simulink library "TYPEBP_MASTER"  (Simulink 8.6)
settings: Solver=ode45  StartTime=0.0  StopTime=10.0  RelTol=1e-3
undefined symbols (not defined in the file): TYPEC, TYPEC_MASTER
libraries: cdsEpicsOut x38, cdsFilt x34, cdsFiltCtrl x24, STATE_BIO_MASTER x18, cdsTP x16, cdsEpicsBinIn x9, VIS_LIB x8, cdsEpicsIn x8, cdsMuxMatrix x5, SIXOSEM_F_STAGE_MASTER x4, cdsEpicsStringIn x3, cdsDacKill x3
(part 2 of 8)

== system TYPEBP_MASTER/TYPEBPMASTER/TEST ==
  In1 : Inport
  In4 : Inport  Port=2
  In7 : Inport  Port=3
  In10 : Inport  Port=4
  CH1 : cdsFiltCtrl/IIR FM with control  Tag=cdsFiltCtrl  Description=|
      | cdsFiltCntrl is the standard IIR filter module (exactly the same as cdsFilt) but with added control data output 'Ctrl'. Filter module digital signal output appears on the first output, which is called 'Val'. 'Ctrl' output has a bit pattern encoding the state of filter's on/off switches (FM1 through FM10). The bit values are:
      |                                                                                                                                                                                                                                                                                                                                       
      | module 	hex	dec                                                                                                                                                                                                                                                                                                                       
      | -----------------------                                                                                                                                                                                                                                                                                                               
      | FM1	0x20                    32                                                                                                                                                                                                                                                                                                        
      | FM2	0x80                     128                                                                                                                                                                                                                                                                                                      
      | FM3	0x200                   512                                                                                                                                                                                                                                                                                                       
      | FM4	0x800                   2048                                                                                                                                                                                                                                                                                                      
      | FM5	0x2000                 8192                                                                                                                                                                                                                                                                                                       
      | FM6	0x8000                 32768                                                                                                                                                                                                                                                                                                      
      | FM7	0x20000                131072                                                                                                                                                                                                                                                                                                     
      | FM8	0x80000                 524288                                                                                                                                                                                                                                                                                                    
      | FM9	0x200000               2097152                                                                                                                                                                                                                                                                                                    
      | FM10	0x800000               8388608                                                                                                                                                                                                                                                                                                   
      |                                                                                                                                                                                                                                                                                                                                       
      | This bit data can be used to drive some other switches or it can be output using a binary I/O module.
      settings: AttributesFormatString=%<Tag>
  CH2 : cdsFiltCtrl/IIR FM with control  Tag=cdsFiltCtrl  Description=|
      | cdsFiltCntrl is the standard IIR filter module (exactly the same as cdsFilt) but with added control data output 'Ctrl'. Filter module digital signal output appears on the first output, which is called 'Val'. 'Ctrl' output has a bit pattern encoding the state of filter's on/off switches (FM1 through FM10). The bit values are:
      |                                                                                                                                                                                                                                                                                                                                       
      | module 	hex	dec                                                                                                                                                                                                                                                                                                                       
      | -----------------------                                                                                                                                                                                                                                                                                                               
      | FM1	0x20                    32                                                                                                                                                                                                                                                                                                        
      | FM2	0x80                     128                                                                                                                                                                                                                                                                                                      
      | FM3	0x200                   512                                                                                                                                                                                                                                                                                                       
      | FM4	0x800                   2048                                                                                                                                                                                                                                                                                                      
      | FM5	0x2000                 8192                                                                                                                                                                                                                                                                                                       
      | FM6	0x8000                 32768                                                                                                                                                                                                                                                                                                      
      | FM7	0x20000                131072                                                                                                                                                                                                                                                                                                     
      | FM8	0x80000                 524288                                                                                                                                                                                                                                                                                                    
      | FM9	0x200000               2097152                                                                                                                                                                                                                                                                                                    
      | FM10	0x800000               8388608                                                                                                                                                                                                                                                                                                   
      |                                                                                                                                                                                                                                                                                                                                       
      | This bit data can be used to drive some other switches or it can be output using a binary I/O module.
      settings: AttributesFormatString=%<Tag>
  CH3 : cdsFiltCtrl/IIR FM with control  Tag=cdsFiltCtrl  Description=|
      | cdsFiltCntrl is the standard IIR filter module (exactly the same as cdsFilt) but with added control data output 'Ctrl'. Filter module digital signal output appears on the first output, which is called 'Val'. 'Ctrl' output has a bit pattern encoding the state of filter's on/off switches (FM1 through FM10). The bit values are:
      |                                                                                                                                                                                                                                                                                                                                       
      | module 	hex	dec                                                                                                                                                                                                                                                                                                                       
      | -----------------------                                                                                                                                                                                                                                                                                                               
      | FM1	0x20                    32                                                                                                                                                                                                                                                                                                        
      | FM2	0x80                     128                                                                                                                                                                                                                                                                                                      
      | FM3	0x200                   512                                                                                                                                                                                                                                                                                                       
      | FM4	0x800                   2048                                                                                                                                                                                                                                                                                                      
      | FM5	0x2000                 8192                                                                                                                                                                                                                                                                                                       
      | FM6	0x8000                 32768                                                                                                                                                                                                                                                                                                      
      | FM7	0x20000                131072                                                                                                                                                                                                                                                                                                     
      | FM8	0x80000                 524288                                                                                                                                                                                                                                                                                                    
      | FM9	0x200000               2097152                                                                                                                                                                                                                                                                                                    
      | FM10	0x800000               8388608                                                                                                                                                                                                                                                                                                   
      |                                                                                                                                                                                                                                                                                                                                       
      | This bit data can be used to drive some other switches or it can be output using a binary I/O module.
      settings: AttributesFormatString=%<Tag>
  CH4 : cdsFiltCtrl/IIR FM with control  Tag=cdsFiltCtrl  Description=|
      | cdsFiltCntrl is the standard IIR filter module (exactly the same as cdsFilt) but with added control data output 'Ctrl'. Filter module digital signal output appears on the first output, which is called 'Val'. 'Ctrl' output has a bit pattern encoding the state of filter's on/off switches (FM1 through FM10). The bit values are:
      |                                                                                                                                                                                                                                                                                                                                       
      | module 	hex	dec                                                                                                                                                                                                                                                                                                                       
      | -----------------------                                                                                                                                                                                                                                                                                                               
      | FM1	0x20                    32                                                                                                                                                                                                                                                                                                        
      | FM2	0x80                     128                                                                                                                                                                                                                                                                                                      
      | FM3	0x200                   512                                                                                                                                                                                                                                                                                                       
      | FM4	0x800                   2048                                                                                                                                                                                                                                                                                                      
      | FM5	0x2000                 8192                                                                                                                                                                                                                                                                                                       
      | FM6	0x8000                 32768                                                                                                                                                                                                                                                                                                      
      | FM7	0x20000                131072                                                                                                                                                                                                                                                                                                     
      | FM8	0x80000                 524288                                                                                                                                                                                                                                                                                                    
      | FM9	0x200000               2097152                                                                                                                                                                                                                                                                                                    
      | FM10	0x800000               8388608                                                                                                                                                                                                                                                                                                   
      |                                                                                                                                                                                                                                                                                                                                       
      | This bit data can be used to drive some other switches or it can be output using a binary I/O module.
      settings: AttributesFormatString=%<Tag>
  Ground{1..6,19,22} (8 alike) : Ground
  Terminator{1..5,16..18} (8 alike) : Terminator
  wires:
  CH1/1 -> Terminator5/1
  CH3/1 -> Terminator3/1
  CH4/1 -> Terminator2/1
  In4/1 -> CH2/1
  CH2/1 -> Terminator4/1
  In1/1 -> CH1/1
  In7/1 -> CH3/1
  In10/1 -> CH4/1
  Ground22/1 -> CH1/2
  Ground19/1 -> CH1/3
  CH1/2 -> Terminator16/1
  CH2/2 -> Terminator17/1
  CH3/2 -> Terminator18/1
  Ground2/1 -> CH2/2
  Ground1/1 -> CH2/3
  Ground4/1 -> CH3/2
  Ground3/1 -> CH3/3
  Ground6/1 -> CH4/2
  Ground5/1 -> CH4/3
  CH4/2 -> Terminator1/1

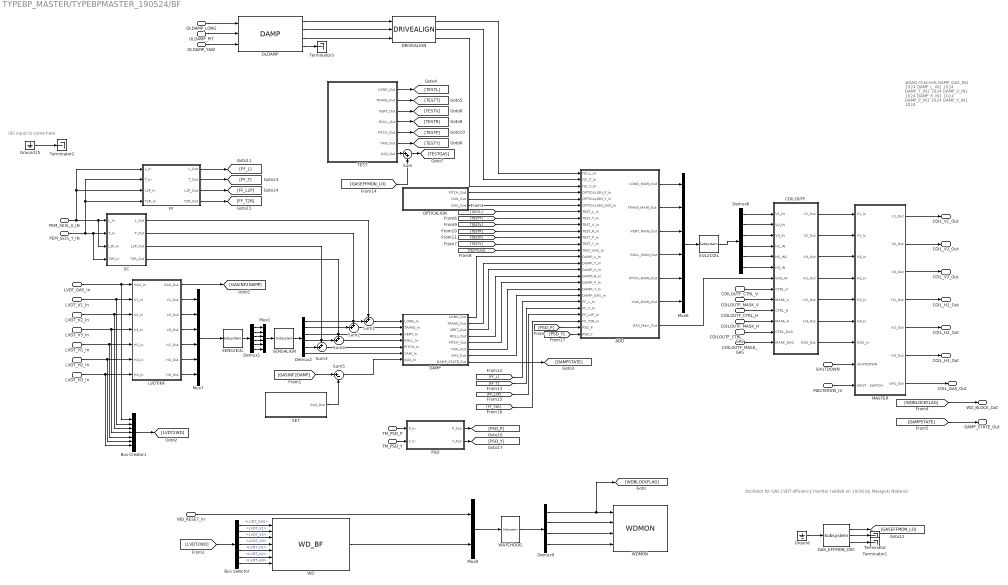
== system TYPEBP_MASTER/TYPEBPMASTER_190524/BF ==
  note: Oscillator for GAS LVDT efficiency monitor (added on 10/26 by Masayuki Nakano)
  note: ISC input to come here
  note: #DAQ Channels
      | DAMP_GAS_IN1 1024
      | DAMP_L_IN1 1024
      | DAMP_T_IN1 1024
      | DAMP_V_IN1 1024
      | DAMP_R_IN1 1024
      | DAMP_P_IN1 1024
      | DAMP_Y_IN1 1024
  LVDT_GAS_In : Inport
  LVDT_V1_In : Inport  Port=2
  LVDT_V2_In : Inport  Port=3
  LVDT_V3_In : Inport  Port=4
  LVDT_H1_In : Inport  Port=5
  LVDT_H2_In : Inport  Port=6
  LVDT_H3_In : Inport  Port=7
  COILOUTF_CTRL_V : Inport  Port=8
  COILOUTF_MASK_V : Inport  Port=9
  COILOUTF_CTRL_H : Inport  Port=10
  COILOUTF_MASK_H : Inport  Port=11
  COILOUTF_CTRL_GAS : Inport  Port=12
  COILOUTF_MASK_GAS : Inport  Port=13
  MASTERSW_In : Inport  Port=14
  WD_RESET_In : Inport  Port=15
  OLDAMP_LONG : Inport  Port=16
  OLDAMP_PIT : Inport  Port=17
  OLDAMP_YAW : Inport  Port=18
  PEM_SEIS_X_IN : Inport  Port=19
  PEM_SEIS_Y_IN : Inport  Port=20
  SHUTDOWN : Inport  Port=21
  TM_PSD_P : Inport  Port=22
  TM_PSD_Y : Inport  Port=23
  ADD : Subsystem
  Bus Creator1 : BusCreator  Inputs='LVDT_GAS','LVDT_V1','LVDT_V2','LVDT_V3','LVDT_H1','LVDT_H2','LVDT_H3'
  Bus Selector : BusSelector  OutputSignals=LVDT_GAS,LVDT_V1,LVDT_V2,LVDT_V3,LVDT_H1,LVDT_H2,LVDT_H3
  COILOUTF : Subsystem
  DAMP : Subsystem
  DRIVEALIGN : VIS_LIB/DRIVEALIGN
  Demux1 : Demux  Outputs=6
  Demux2 : Demux  Outputs=6
  Demux6 : Demux  Outputs=6
  Demux9 : Demux
  EUL2COIL : cdsMuxMatrix/Subsystem  Tag=cdsMuxMatrix  Description=|
      | ADL=SUS_INMATRIX.adl
      | SCRIPT=generate_KisselButton.py 4 5 #CHANNEL# > #TARGET_DIR#/#FULL_PART_NAME#_KB.adl
      settings: AttributesFormatString=%<Tag>
  FF : Subsystem
  GAS_EFFMON_OSC : cdsOsc/Subsystem  Tag=cdsOsc  Description=Oscillator
      settings: AttributesFormatString=%<Tag>
  Ground : Ground
  Ground15 : Ground
  LVDTINF : Subsystem
  MASTER : Subsystem
  Mux1 : Mux  Inputs=6
  Mux6 : Mux  Inputs=6
  Mux7 : Mux  Inputs=6
  Mux9 : Mux  Inputs=2
  OLDAMP : VIS_LIB/DAMP
  OPTICALIGN : Subsystem
  PSD : Subsystem
  SC : Subsystem
  SENS2EUL : cdsMuxMatrix/Subsystem  Tag=cdsMuxMatrix  Description=Any size matrix. Inputs and outputs must be connected using Mux and Demux parts.
      settings: AttributesFormatString=%<Tag>
  SENSALIGN : cdsMuxMatrix/Subsystem  Tag=cdsMuxMatrix  Description=Any size matrix. Inputs and outputs must be connected using Mux and Demux parts.
      settings: AttributesFormatString=%<Tag>
  SET : Subsystem
  Sum : Sum  Inputs=|++
  Sum{1..4} (4 alike) : Sum  Inputs=++|
  Sum5 : Sum  Inputs=|+-
  TEST : Subsystem
  Terminator{,1..3} (4 alike) : Terminator
  WATCHDOG : cdsFunctionCall/Subsystem  Tag=cdsFunctionCall  Description=inline OSEMWATCHDOG /opt/rtcds/userapps/release/vis/common/src/WATCHDOG.c
      settings: AttributesFormatString=%<Tag>\n%<Description>
  WD : VIS_LIB/WD_BF
  WDMON : SIXOSEM_F_STAGE_MASTER/SIXOSEM_F_STAGE_MASTER/WDMON
  COIL_GAS_Out : Outport
  COIL_V1_Out : Outport  Port=2
  COIL_V2_Out : Outport  Port=3
  COIL_V3_Out : Outport  Port=4
  COIL_H1_Out : Outport  Port=5
  COIL_H2_Out : Outport  Port=6
  COIL_H3_Out : Outport  Port=7
  WD_BLOCK_Out : Outport  Port=8
  DAMP_STATE_Out : Outport  Port=9
  wires:
  PSD/2(Y_Out) -> [PSD_Y]
  PSD/1(P_Out) -> [PSD_P]
  TM_PSD_Y/1 -> PSD/2(Y_In)
  TM_PSD_P/1 -> PSD/1(P_In)
  [PSD_Y] -> ADD/26(PSD_Y)
  [PSD_P] -> ADD/25(PSD_P)
  Mux7/1 -> SENS2EUL/1
  Mux6/1 -> EUL2COIL/1
  EUL2COIL/1 -> Demux6/1
  MASTER/1(V1_Out) -> COIL_V1_Out/1
  MASTER/2(V2_Out) -> COIL_V2_Out/1
  MASTER/3(V3_Out) -> COIL_V3_Out/1
  WD_RESET_In/1 -> Mux9/1
  WD/1 -> Mux9/2
  [LVDT2WD] -> Bus Selector/1
  Demux9/1 -> [WDBLOCKFLAG], WDMON/1
  Demux9/2 -> WDMON/2
  Demux9/3 -> WDMON/3
  Demux9/4 -> WDMON/4
  Mux9/1 -> WATCHDOG/1
  WATCHDOG/1 -> Demux9/1
  LVDT_V1_In/1 -> Bus Creator1/2, LVDTINF/2(V1_In)
  LVDT_V2_In/1 -> Bus Creator1/3, LVDTINF/3(V2_In)
  LVDT_V3_In/1 -> Bus Creator1/4, LVDTINF/4(V3_In)
  LVDT_H1_In/1 -> LVDTINF/5(H1_In), Bus Creator1/5
  LVDT_H2_In/1 -> LVDTINF/6(H2_In), Bus Creator1/6
  LVDT_H3_In/1 -> LVDTINF/7(H3_In), Bus Creator1/7
  Bus Creator1/1 -> [LVDT2WD]
  COILOUTF_CTRL_V/1 -> COILOUTF/8(CTRL_V)
  COILOUTF_MASK_V/1 -> COILOUTF/9(MASK_V)
  LVDT_GAS_In/1 -> Bus Creator1/1, LVDTINF/1(GAS_In)
  LVDTINF/1(GAS_Out) -> [GASINF2DAMP]
  TEST/1(LONG_Out) -> [TESTL]
  TEST/2(TRANS_Out) -> [TESTT]
  TEST/6(YAW_Out) -> [TESTY]
  [TESTL] -> ADD/7(TEST_L_In)
  [TESTT] -> ADD/8(TEST_T_In)
  [TESTY] -> ADD/12(TEST_Y_In)
  [TESTGAS] -> ADD/13(TEST_GAS_In)
  MASTER/4(H1_Out) -> COIL_H1_Out/1
  Bus Selector/1 -> WD/1  "<LVDT_GAS>"
  Demux2/6 -> DAMP/6(YAW_In)
  Demux2/5 -> Sum3/2
  Demux2/4 -> Sum4/2
  Demux2/3 -> DAMP/3(VERT_In)
  Demux2/2 -> Sum2/2
  Demux2/1 -> Sum1/2
  SENS2EUL/1 -> Demux1/1
  Demux1/1 -> Mux1/1
  Demux1/2 -> Mux1/2
  Demux1/3 -> Mux1/3
  Demux1/4 -> Mux1/4
  Demux1/5 -> Mux1/5
  Demux1/6 -> Mux1/6
  Mux1/1 -> SENSALIGN/1
  SENSALIGN/1 -> Demux2/1
  LVDTINF/2(V1_Out) -> Mux7/1
  LVDTINF/3(V2_Out) -> Mux7/2
  LVDTINF/4(V3_Out) -> Mux7/3
  DAMP/8(DAMP_STATE_Out) -> [DAMPSTATE]
  TEST/3(VERT_Out) -> [TESTV]
  TEST/4(ROLL_Out) -> [TESTR]
  TEST/5(PITCH_Out) -> [TESTP]
  [TESTV] -> ADD/9(TEST_V_In)
  [TESTR] -> ADD/10(TEST_R_In)
  [TESTP] -> ADD/11(TEST_P_In)
  DAMP/7(GAS_Out) -> ADD/20(DAMP_GAS_In)
  DAMP/6(YAW_Out) -> ADD/19(DAMP_Y_In)
  DAMP/5(PITCH_Out) -> ADD/18(DAMP_P_In)
  DAMP/4(ROLL_Out) -> ADD/17(DAMP_R_In)
  DAMP/3(VERT_Out) -> ADD/16(DAMP_V_In)
  DAMP/2(TRANS_Out) -> ADD/15(DAMP_T_In)
  DAMP/1(LONG_Out) -> ADD/14(DAMP_L_In)
  ADD/7(GAS_Main_Out) -> COILOUTF/7(GAS_IN)
  ADD/6(YAW_MAIN_Out) -> Mux6/6
  ADD/5(PITCH_MAIN_Out) -> Mux6/5
  ADD/4(ROLL_MAIN_Out) -> Mux6/4
  ADD/3(VERT_MAIN_Out) -> Mux6/3
  ADD/2(TRANS_MAIN_Out) -> Mux6/2
  ADD/1(LONG_MAIN_Out) -> Mux6/1
  OPTICALIGN/1(PITCH_Out) -> ADD/4(OPTICALIGN_P_In)
  OPTICALIGN/2(YAW_Out) -> ADD/5(OPTICALIGN_Y_In)
  OPTICALIGN/3(GAS_Out) -> ADD/6(OPTICALIGN_GAS_In)
  Demux6/1 -> COILOUTF/1(V1_IN)
  Demux6/2 -> COILOUTF/2(V2_IN)
  Demux6/3 -> COILOUTF/3(V3_IN)
  Demux6/4 -> COILOUTF/4(H1_IN)
  Demux6/5 -> COILOUTF/5(H2_IN1)
  Demux6/6 -> COILOUTF/6(H3_IN)
  COILOUTF/5(H2_Out) -> MASTER/5(H2_In)
  COILOUTF/6(H3_Out) -> MASTER/6(H3_In)
  COILOUTF/7(GAS_Out) -> MASTER/7(GAS_In)
  COILOUTF/1(V1_Out) -> MASTER/1(V1_In)
  COILOUTF/2(V2_Out) -> MASTER/2(V2_In)
  COILOUTF/3(V3_Out) -> MASTER/3(V3_In)
  COILOUTF/4(H1_Out) -> MASTER/4(H1_In)
  SHUTDOWN/1 -> MASTER/8(SHUTDOWN)
  MASTERSW_In/1 -> MASTER/9(MASTERSWITCH)
  MASTER/5(H2_Out) -> COIL_H2_Out/1
  MASTER/6(H3_Out) -> COIL_H3_Out/1
  MASTER/7(GAS_Out) -> COIL_GAS_Out/1
  [WDBLOCKFLAG] -> WD_BLOCK_Out/1
  [DAMPSTATE] -> DAMP_STATE_Out/1
  Bus Selector/2 -> WD/2  "<LVDT_V1>"
  Bus Selector/3 -> WD/3  "<LVDT_V2>"
  Bus Selector/4 -> WD/4  "<LVDT_V3>"
  Bus Selector/5 -> WD/5  "<LVDT_H1>"
  Bus Selector/6 -> WD/6  "<LVDT_H2>"
  Bus Selector/7 -> WD/7  "<LVDT_H3>"
  LVDTINF/5(H1_Out) -> Mux7/4
  LVDTINF/6(H2_Out) -> Mux7/5
  LVDTINF/7(H3_Out) -> Mux7/6
  COILOUTF_CTRL_H/1 -> COILOUTF/10(CTRL_H)
  COILOUTF_MASK_H/1 -> COILOUTF/11(MASK_H)
  COILOUTF_CTRL_GAS/1 -> COILOUTF/12(CTRL_GAS)
  COILOUTF_MASK_GAS/1 -> COILOUTF/13(MASK_GAS)
  GAS_EFFMON_OSC/1 -> [GASEFFMON_LO]
  TEST/7(GAS_Out) -> Sum/1
  Sum/1 -> [TESTGAS]
  [GASEFFMON_LO] -> Sum/2
  Ground/1 -> GAS_EFFMON_OSC/1
  GAS_EFFMON_OSC/2 -> Terminator/1
  GAS_EFFMON_OSC/3 -> Terminator1/1
  OLDAMP/4 -> Terminator3/1
  OLDAMP_YAW/1 -> OLDAMP/3
  OLDAMP_PIT/1 -> OLDAMP/2
  OLDAMP_LONG/1 -> OLDAMP/1
  Ground15/1 -> Terminator2/1
  OLDAMP/1 -> DRIVEALIGN/1
  OLDAMP/2 -> DRIVEALIGN/2
  OLDAMP/3 -> DRIVEALIGN/3
  DRIVEALIGN/3 -> ADD/3(ISC_Y_In)
  DRIVEALIGN/2 -> ADD/2(ISC_P_In)
  DRIVEALIGN/1 -> ADD/1(ISC_L_In)
  SC/1(L_Out) -> Sum1/1
  PEM_SEIS_Y_IN/1 -> SC/4(T2R_In), SC/2(T_In), FF/4(T2R_In), FF/2(T_In)
  SC/2(T_Out) -> Sum2/1
  Sum1/1 -> DAMP/1(LONG_In)
  Sum2/1 -> DAMP/2(TRANS_In)
  PEM_SEIS_X_IN/1 -> FF/1(L_In), FF/3(L2P_In), SC/3(L2P_In), SC/1(L_In)
  FF/1(L_Out) -> [FF_L]
  FF/2(T_Out) -> [FF_T]
  [FF_L] -> ADD/21(FF_L_In)
  [FF_T] -> ADD/22(FF_T_In)
  FF/3(L2P_Out) -> [FF_L2P]
  FF/4(T2R_Out) -> [FF_T2R]
  [FF_L2P] -> ADD/23(FF_L2P_In)
  [FF_T2R] -> ADD/24(FF_T2R_In)
  Sum3/1 -> DAMP/5(PITCH_In)
  SC/3(L2P_Out) -> Sum3/1
  Sum4/1 -> DAMP/4(ROLL_In)
  SC/4(T2R_Out) -> Sum4/1
  [GASINF2DAMP] -> Sum5/1
  Sum5/1 -> DAMP/7(GAS_In)
  SET/1(GAS_Out) -> Sum5/2

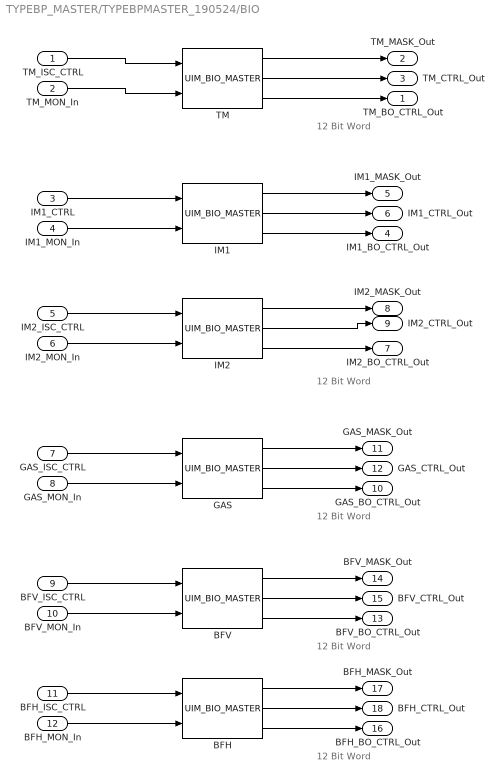
== system TYPEBP_MASTER/TYPEBPMASTER_190524/BIO ==
  note: 12 Bit Word
  note: 12 Bit Word
  note: 12 Bit Word
  note: 12 Bit Word
  note: 12 Bit Word
  TM_ISC_CTRL : Inport
  TM_MON_In : Inport  Port=2
  IM1_CTRL : Inport  Port=3
  IM1_MON_In : Inport  Port=4
  IM2_ISC_CTRL : Inport  Port=5
  IM2_MON_In : Inport  Port=6
  GAS_ISC_CTRL : Inport  Port=7
  GAS_MON_In : Inport  Port=8
  BFV_ISC_CTRL : Inport  Port=9
  BFV_MON_In : Inport  Port=10
  BFH_ISC_CTRL : Inport  Port=11
  BFH_MON_In : Inport  Port=12
  BFH : STATE_BIO_MASTER/UIM_BIO_MASTER
  BFV : STATE_BIO_MASTER/UIM_BIO_MASTER
  GAS : STATE_BIO_MASTER/UIM_BIO_MASTER
  IM1 : STATE_BIO_MASTER/UIM_BIO_MASTER
  IM2 : STATE_BIO_MASTER/UIM_BIO_MASTER
  TM : STATE_BIO_MASTER/UIM_BIO_MASTER
  TM_BO_CTRL_Out : Outport
  TM_MASK_Out : Outport  Port=2
  TM_CTRL_Out : Outport  Port=3
  IM1_BO_CTRL_Out : Outport  Port=4
  IM1_MASK_Out : Outport  Port=5
  IM1_CTRL_Out : Outport  Port=6
  IM2_BO_CTRL_Out : Outport  Port=7
  IM2_MASK_Out : Outport  Port=8
  IM2_CTRL_Out : Outport  Port=9
  GAS_BO_CTRL_Out : Outport  Port=10
  GAS_MASK_Out : Outport  Port=11
  GAS_CTRL_Out : Outport  Port=12
  BFV_BO_CTRL_Out : Outport  Port=13
  BFV_MASK_Out : Outport  Port=14
  BFV_CTRL_Out : Outport  Port=15
  BFH_BO_CTRL_Out : Outport  Port=16
  BFH_MASK_Out : Outport  Port=17
  BFH_CTRL_Out : Outport  Port=18
  wires:
  BFV/3 -> BFV_BO_CTRL_Out/1
  BFV/2 -> BFV_CTRL_Out/1
  BFV/1 -> BFV_MASK_Out/1
  GAS/3 -> GAS_BO_CTRL_Out/1
  GAS/2 -> GAS_CTRL_Out/1
  GAS/1 -> GAS_MASK_Out/1
  IM2/3 -> IM2_BO_CTRL_Out/1
  IM2/2 -> IM2_CTRL_Out/1
  IM2/1 -> IM2_MASK_Out/1
  IM1/3 -> IM1_BO_CTRL_Out/1
  IM1/2 -> IM1_CTRL_Out/1
  IM1/1 -> IM1_MASK_Out/1
  TM/3 -> TM_BO_CTRL_Out/1
  TM/2 -> TM_CTRL_Out/1
  TM/1 -> TM_MASK_Out/1
  BFV_ISC_CTRL/1 -> BFV/1
  BFV_MON_In/1 -> BFV/2
  GAS_ISC_CTRL/1 -> GAS/1
  GAS_MON_In/1 -> GAS/2
  IM2_ISC_CTRL/1 -> IM2/1
  IM2_MON_In/1 -> IM2/2
  IM1_MON_In/1 -> IM1/2
  IM1_CTRL/1 -> IM1/1
  TM_ISC_CTRL/1 -> TM/1
  TM_MON_In/1 -> TM/2
  BFH/3 -> BFH_BO_CTRL_Out/1
  BFH/2 -> BFH_CTRL_Out/1
  BFH/1 -> BFH_MASK_Out/1
  BFH_ISC_CTRL/1 -> BFH/1
  BFH_MON_In/1 -> BFH/2

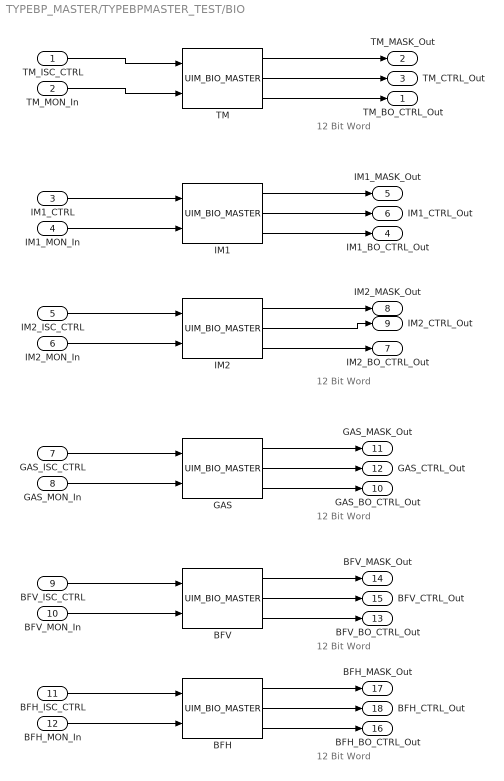
== system TYPEBP_MASTER/TYPEBPMASTER_TEST/BIO ==
  note: 12 Bit Word
  note: 12 Bit Word
  note: 12 Bit Word
  note: 12 Bit Word
  note: 12 Bit Word
  TM_ISC_CTRL : Inport
  TM_MON_In : Inport  Port=2
  IM1_CTRL : Inport  Port=3
  IM1_MON_In : Inport  Port=4
  IM2_ISC_CTRL : Inport  Port=5
  IM2_MON_In : Inport  Port=6
  GAS_ISC_CTRL : Inport  Port=7
  GAS_MON_In : Inport  Port=8
  BFV_ISC_CTRL : Inport  Port=9
  BFV_MON_In : Inport  Port=10
  BFH_ISC_CTRL : Inport  Port=11
  BFH_MON_In : Inport  Port=12
  BFH : STATE_BIO_MASTER/UIM_BIO_MASTER
  BFV : STATE_BIO_MASTER/UIM_BIO_MASTER
  GAS : STATE_BIO_MASTER/UIM_BIO_MASTER
  IM1 : STATE_BIO_MASTER/UIM_BIO_MASTER
  IM2 : STATE_BIO_MASTER/UIM_BIO_MASTER
  TM : STATE_BIO_MASTER/UIM_BIO_MASTER
  TM_BO_CTRL_Out : Outport
  TM_MASK_Out : Outport  Port=2
  TM_CTRL_Out : Outport  Port=3
  IM1_BO_CTRL_Out : Outport  Port=4
  IM1_MASK_Out : Outport  Port=5
  IM1_CTRL_Out : Outport  Port=6
  IM2_BO_CTRL_Out : Outport  Port=7
  IM2_MASK_Out : Outport  Port=8
  IM2_CTRL_Out : Outport  Port=9
  GAS_BO_CTRL_Out : Outport  Port=10
  GAS_MASK_Out : Outport  Port=11
  GAS_CTRL_Out : Outport  Port=12
  BFV_BO_CTRL_Out : Outport  Port=13
  BFV_MASK_Out : Outport  Port=14
  BFV_CTRL_Out : Outport  Port=15
  BFH_BO_CTRL_Out : Outport  Port=16
  BFH_MASK_Out : Outport  Port=17
  BFH_CTRL_Out : Outport  Port=18
  wires:
  BFH_MON_In/1 -> BFH/2
  BFH_ISC_CTRL/1 -> BFH/1
  BFH/1 -> BFH_MASK_Out/1
  BFH/2 -> BFH_CTRL_Out/1
  BFH/3 -> BFH_BO_CTRL_Out/1
  TM_MON_In/1 -> TM/2
  TM_ISC_CTRL/1 -> TM/1
  IM1_CTRL/1 -> IM1/1
  IM1_MON_In/1 -> IM1/2
  IM2_MON_In/1 -> IM2/2
  IM2_ISC_CTRL/1 -> IM2/1
  GAS_MON_In/1 -> GAS/2
  GAS_ISC_CTRL/1 -> GAS/1
  BFV_MON_In/1 -> BFV/2
  BFV_ISC_CTRL/1 -> BFV/1
  TM/1 -> TM_MASK_Out/1
  TM/2 -> TM_CTRL_Out/1
  TM/3 -> TM_BO_CTRL_Out/1
  IM1/1 -> IM1_MASK_Out/1
  IM1/2 -> IM1_CTRL_Out/1
  IM1/3 -> IM1_BO_CTRL_Out/1
  IM2/1 -> IM2_MASK_Out/1
  IM2/2 -> IM2_CTRL_Out/1
  IM2/3 -> IM2_BO_CTRL_Out/1
  GAS/1 -> GAS_MASK_Out/1
  GAS/2 -> GAS_CTRL_Out/1
  GAS/3 -> GAS_BO_CTRL_Out/1
  BFV/1 -> BFV_MASK_Out/1
  BFV/2 -> BFV_CTRL_Out/1
  BFV/3 -> BFV_BO_CTRL_Out/1

== system TYPEBP_MASTER/TYPEBPMASTER_TEST/SF ==
  note: #DAQ Channels
      | LVDTINF_GAS_IN1 2048
      | DAMP_GAS_IN1 2048
  LVDT_GAS_IN : Inport
  COILOUT_CTRL : Inport  Port=2
  COILOUTF_MASK : Inport  Port=3
  MASTERSW_IN : Inport  Port=4
  WDRESET_IN : Inport  Port=5
  PEM_SEIS_Z_IN : Inport  Port=6
  ADD : Subsystem
  COILOUTF : Subsystem
  DAMP : Subsystem
  Demux9 : Demux
  FF : Subsystem
  LVDTINF : Subsystem
  MASTER : Subsystem
  Mux9 : Mux  Inputs=2
  SC : Subsystem
  Sum : Sum  Inputs=++|
  TEST : Subsystem
  WATCHDOG : cdsFunctionCall/Subsystem  Tag=cdsFunctionCall  Description=inline OSEMWATCHDOG /opt/rtcds/userapps/release/vis/common/src/WATCHDOG.c
      settings: AttributesFormatString=%<Tag>\n%<Description>
  WD : VIS_LIB/WD_GAS
  WDMON : VIS_LIB/WDMON
  GAS_CTR_OUT : Outport
  WD_STAT_OUT : Outport  Port=2
  DAMP_STAT_OUT : Outport  Port=3
  wires:
  Demux9/2 -> WDMON/2
  Demux9/3 -> WDMON/3
  WD/1 -> Mux9/2
  COILOUTF/1(Out1) -> MASTER/1(GAS_In)
  LVDTINF/1(Out1) -> Sum/2
  WATCHDOG/1 -> Demux9/1
  Demux9/4 -> WDMON/4
  Mux9/1 -> WATCHDOG/1
  DAMP/2(DAMP_STATE_Out) -> [DAMPSTATE]
  DAMP/1(F0_Out) -> ADD/3(DAMP_In)
  MASTERSW_IN/1 -> MASTER/2(MASTERSWITCH)
  [WDBLOCKFLAG] -> WD_STAT_OUT/1
  [DAMPSTATE] -> DAMP_STAT_OUT/1
  TEST/1(F0_Out) -> ADD/2(TEST_In)
  [WDBLOCKFLAG] -> MASTER/3(WDFLAG)
  MASTER/1(GAS_Out) -> GAS_CTR_OUT/1
  ADD/1(GAS_MAIN_Out) -> COILOUTF/1(In1)
  Demux9/1 -> [WDBLOCKFLAG], WDMON/1
  LVDT_GAS_IN/1 -> LVDTINF/1(In1), WD/1
  COILOUT_CTRL/1 -> COILOUTF/2(In2)
  COILOUTF_MASK/1 -> COILOUTF/3(In3)
  WDRESET_IN/1 -> Mux9/1
  PEM_SEIS_Z_IN/1 -> FF/1(In1), SC/1(In1)
  SC/1(Out1) -> Sum/1
  Sum/1 -> DAMP/1(GAS_In)
  FF/1(Out1) -> ADD/1(FF_In)
